simulink model "DC_Motor_Dynamic_Model"  (R2021a)
settings: Solver=VariableStepAuto  StartTime=0.0  StopTime=10  RelTol=1e-3
InitFcn:
  | Kf=.8;
  | TL=0;
  | 
  | Ra=1.43;
  | La=10.4*10^(-3);
  | 
  | Rf=5;
  | Lf=2;
  | 
  | Maf=1.8;
  | 
  | j=.068;
  | B=0;
settings Model: Creator=User  LastModifiedBy=User
settings SolverCC: AlgebraicLoopSolver=TrustRegion
settings DebuggingCC: SFMachineParentedDataDiag=warning

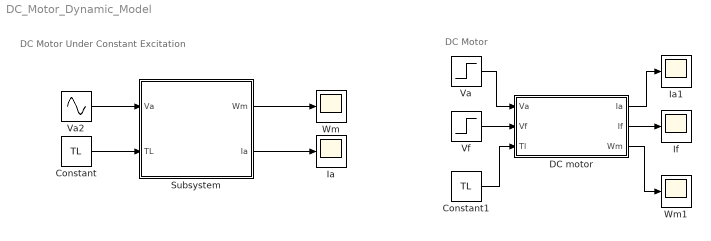
== system DC_Motor_Dynamic_Model ==
  note: DC Motor
  note: DC Motor Under Constant Excitation
  Constant : Constant  Value=TL
  Constant1 : Constant  Value=TL
  DC motor : Subsystem
  Ia : Scope
  Ia1 : Scope
  If : Scope
  Subsystem : Subsystem
  Va : Step  After=240  SampleTime=0
  Va2 : Sin  Amplitude=200  SampleTime=0
  Vf : Step  Before=5  After=5  SampleTime=0
  Wm : Scope
  Wm1 : Scope
  wires:
  Constant/1 -> Subsystem/2(TL)
  Va2/1 -> Subsystem/1(Va)
  Subsystem/1(Wm) -> Wm/1
  Subsystem/2(Ia) -> Ia/1
  Constant1/1 -> DC motor/3(Tl)
  Va/1 -> DC motor/1(Va)
  DC motor/3(Wm) -> Wm1/1
  DC motor/1(Ia) -> Ia1/1
  DC motor/2(If) -> If/1
  Vf/1 -> DC motor/2(Vf)

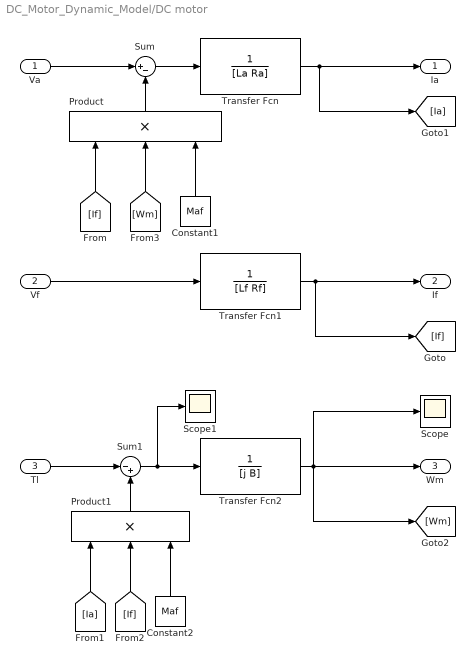
== system DC_Motor_Dynamic_Model/DC motor ==
  Va : Inport
  Vf : Inport  Port=2
  Tl : Inport  Port=3
  Constant1 : Constant  Value=Maf
  Constant2 : Constant  Value=Maf
  Product : Product  Inputs=3
  Product1 : Product  Inputs=3
  Scope : Scope
  Scope1 : Scope
  Sum : Sum  Inputs=|+-
  Sum1 : Sum  Inputs=|-+
  Transfer Fcn : TransferFcn  Denominator=[La Ra]
  Transfer Fcn1 : TransferFcn  Denominator=[Lf Rf]
  Transfer Fcn2 : TransferFcn  Denominator=[j B]
  Ia : Outport
  If : Outport  Port=2
  Wm : Outport  Port=3
  wires:
  Transfer Fcn/1 -> Ia/1, [Ia]
  Product1/1 -> Sum1/2
  Vf/1 -> Transfer Fcn1/1
  Product/1 -> Sum/2
  Sum1/1 -> Scope1/1, Transfer Fcn2/1
  Transfer Fcn1/1 -> If/1, [If]
  Transfer Fcn2/1 -> Wm/1, [Wm], Scope/1
  Va/1 -> Sum/1
  Sum/1 -> Transfer Fcn/1
  [Ia] -> Product1/1
  [Wm] -> Product/2
  [If] -> Product1/2
  Tl/1 -> Sum1/1
  [If] -> Product/1
  Constant2/1 -> Product1/3
  Constant1/1 -> Product/3

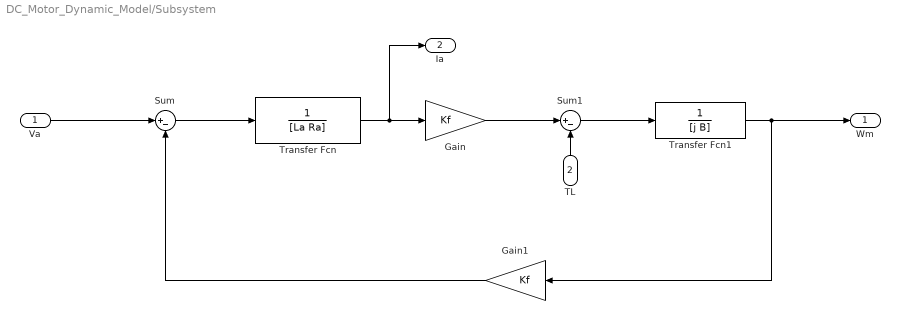
== system DC_Motor_Dynamic_Model/Subsystem ==
  Va : Inport
  TL : Inport  Port=2
  Gain : Gain  Gain=Kf
  Gain1 : Gain  Gain=Kf
  Sum : Sum  Inputs=|+-
  Sum1 : Sum  Inputs=|+-
  Transfer Fcn : TransferFcn  Denominator=[La Ra]
  Transfer Fcn1 : TransferFcn  Denominator=[j B]
  Wm : Outport
  Ia : Outport  Port=2
  wires:
  Gain1/1 -> Sum/2
  Sum/1 -> Transfer Fcn/1
  Transfer Fcn1/1 -> Wm/1, Gain1/1
  TL/1 -> Sum1/2
  Transfer Fcn/1 -> Ia/1, Gain/1
  Sum1/1 -> Transfer Fcn1/1
  Gain/1 -> Sum1/1
  Va/1 -> Sum/1
